simulink model "audio_test_1"  (Simulink 7.8)
settings: Solver=ode45  StartTime=0.0  StopTime=1  RelTol=1e-3
values from neighbouring files (symbols this model uses):
  a1 = 2    [audio_test1.m]    (also in audio_test2.m)
  a2 = 3    [audio_test1.m]    (also in audio_test2.m)
  f1 = 0.1    [CFIR_1.m]    (also in analog_bp1.m = ',num2str(f1),' Hz; analog_bp11.m = ',num2str(f1),' Hz; analog_bp2.m = 30000; analog_bp3.m = 30000)
  f2 = 0.3    [CFIR_1.m]    (also in analog_bp1.m = ',num2str(f2),' Hz)']); analog_bp11.m = ',num2str(f2),' Hz)']); analog_bp2.m = 35000; analog_bp3.m = 30500)
  g0t = g0'    [audio_test1.m]    (also in audio_test2.m)
  g1t = g1'    [audio_test1.m]    (also in audio_test2.m)
  h0t = h0'    [audio_test1.m]    (also in audio_test2.m)
  h1t = h1'    [audio_test1.m]    (also in audio_test2.m)
  L = 24    [G722_1.m]    (also in adaptiv_2.m = length(h); adaptiv_3.m = length(h); audio_test1.m = 64; audio_test2.m = 64)
  Ts = 1/fs    (= 6.25e-05)    [G722_1.m]    (also in adaptiv_2.m = 0.001; adaptiv_3.m = 0.001; adaptiv_4.m = 0.001; adaptiv_5.m = 0.001)
undefined symbols (not defined in the file or in its folder): get, One, sided
libraries: dspsnks4 x7, dspsigops x5
settings Model: Creator=svenhoffmann  LastModifiedBy=josef  ExtModeAutoUpdateStatusClock=off
settings DataIOCC: SignalLoggingName=sigsOut
settings OptimizationCC: InitFltsAndDblsToZero=on
settings DebuggingCC: SaveWithParameterizedLinksMsg=none  SignalResolutionControl=TryResolveAllWithWarning  SolverPrmCheckMsg=none  MultiTaskDSMMsg=warning  MultiTaskCondExecSysMsg=none  FcnCallInpInsideContextMsg=Use local settings  StrictBusMsg=None
settings HardwareCC: TargetUnknown=on
settings RTWCC: IncludeERTFirstTime=on
settings GRTTargetCC: TargetFcnLib=ansi_tfl_tmw.mat

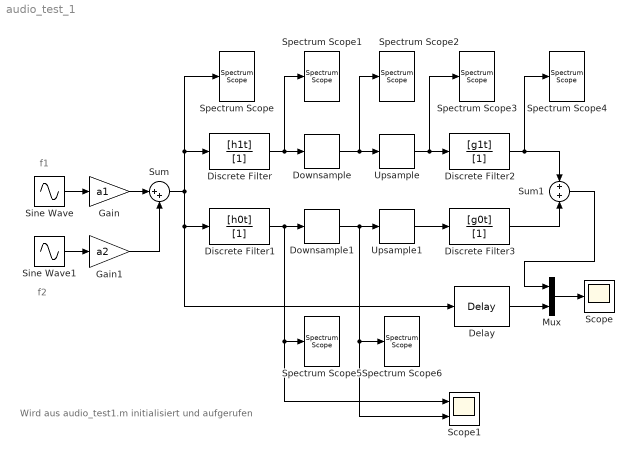
== system audio_test_1 ==
  note: f1
  note: f2
  note: Wird aus audio_test1.m initialisiert und aufgerufen
  Delay : dspsigops/Delay  InputProcessing=Inherited (this choice will be removed - see release notes)  dly_unit=Samples  delay=L-1  ic_detail=off  dif_ic_for_ch=off  dif_ic_for_dly=off  ic=0  reset_popup=None
  Discrete Filter : DiscreteFilter  Numerator=[h1t]  Denominator=[1]  SampleTime=Ts
  Discrete Filter1 : DiscreteFilter  Numerator=[h0t]  Denominator=[1]  SampleTime=Ts
  Discrete Filter2 : DiscreteFilter  Numerator=[g1t]  Denominator=[1]  SampleTime=Ts
  Discrete Filter3 : DiscreteFilter  Numerator=[g0t]  Denominator=[1]  SampleTime=Ts
  Downsample : dspsigops/Downsample  N=2  phase=0  InputProcessing=Inherited (this choice will be removed - see release notes)  RateOptions=Enforce single-rate processing  smode=Allow multirate  fmode=Maintain input frame size  ic=0
  Downsample1 : dspsigops/Downsample  N=2  phase=0  InputProcessing=Inherited (this choice will be removed - see release notes)  RateOptions=Enforce single-rate processing  smode=Allow multirate  fmode=Maintain input frame size  ic=0
  Gain : Gain  Gain=a1  SaturateOnIntegerOverflow=on  OutDataTypeStr=Inherit: Same as input  ParamDataTypeStr=Inherit: Same as input
  Gain1 : Gain  Gain=a2  SaturateOnIntegerOverflow=on  OutDataTypeStr=Inherit: Same as input  ParamDataTypeStr=Inherit: Same as input
  Mux : Mux  Inputs=2
  Scope : Scope
  Scope1 : Scope  NumInputPorts=2
      settings: YMin=-5~-5  YMax=5~5
  Sine Wave : Sin  Frequency=2*pi*f1  SampleTime=Ts
  Sine Wave1 : Sin  Frequency=2*pi*f2  SampleTime=Ts
  Spectrum Scope{,1..6} (7 alike) : dspsnks4/Spectrum Scope  ScopeProperties=on  Domain=Frequency  HorizSpan=1  UseBuffer=on  BufferSize=256  Overlap=0  TreatMby1Signals=M channels  inpFftLenInherit=on  FFTlength=256  numAvg=5  DisplayProperties=off  AxisGrid=on  Memory=off  FrameNumber=on  AxisLegend=off  AxisZoom=off  OpenScopeAtSimStart=on  OpenScopeImmediately=off  FigPos=get(0,'defaultfigureposition')  AxisProperties=off  XUnits=Hertz  XRange=One-sided ([0...Fs/2])  XDisplay=0  InheritXIncr=on  XIncr=1.0  XLabel=Samples  XLimit=Auto  YUnits=dBW/Hertz  XMax=1  XMin=0  YLabel=Magnitude, dB  LineProperties=off  wintypeSpecScope=Hann  RsSpecScope=50  betaSpecScope=5  winsampSpecScope=Periodic  XAxisParamsVer=6.8  isFrameUpgraded=on
      Spectrum Scope settings: YMin=-93.3851382327638  YMax=26.8995971188015
      Spectrum Scope1 settings: YMin=-109.465065113962  YMax=30.059546519903
      Spectrum Scope2 settings: YMin=-107.176539343052  YMax=29.3444879435202
      Spectrum Scope3 settings: YMin=-98.918847369225  YMax=23.7379166188996
      Spectrum Scope4 settings: YMin=-117.083304354363  YMax=26.8978660120825
      Spectrum Scope5 settings: YMin=-117.083304354363  YMax=26.8978660120825
      Spectrum Scope6 settings: YMin=-117.083304354363  YMax=26.8978660120825
  Sum : Sum  Inputs=|++  SaturateOnIntegerOverflow=on
  Sum1 : Sum  SaturateOnIntegerOverflow=on
  Upsample : dspsigops/Upsample  N=2  phase=0  InputProcessing=Inherited (this choice will be removed - see release notes)  RateOptions=Allow multirate processing  ic=0  mode=Unused parameter value
  Upsample1 : dspsigops/Upsample  N=2  phase=0  InputProcessing=Inherited (this choice will be removed - see release notes)  RateOptions=Allow multirate processing  ic=0  mode=Unused parameter value
  wires:
  Sine Wave/1 -> Gain/1
  Sine Wave1/1 -> Gain1/1
  Gain/1 -> Sum/1
  Gain1/1 -> Sum/2
  Sum/1 -> Discrete Filter1/1, Delay/1, Discrete Filter/1, Spectrum Scope/1
  Discrete Filter/1 -> Downsample/1, Spectrum Scope1/1
  Discrete Filter1/1 -> Downsample1/1, Spectrum Scope5/1, Scope1/1
  Downsample/1 -> Upsample/1, Spectrum Scope2/1
  Downsample1/1 -> Upsample1/1, Spectrum Scope6/1, Scope1/2
  Upsample/1 -> Discrete Filter2/1, Spectrum Scope3/1
  Upsample1/1 -> Discrete Filter3/1
  Discrete Filter2/1 -> Sum1/1, Spectrum Scope4/1
  Discrete Filter3/1 -> Sum1/2
  Mux/1 -> Scope/1
  Sum1/1 -> Mux/1
  Delay/1 -> Mux/2
